simulink model "cruise_control_external_sfun"  (R2013a)
settings: Solver=ode1  StartTime=0.0  StopTime=inf  FixedStep=0.1  RelTol=1e-3
PreLoadFcn:
  | load('cruise_control_external.mat')
undefined symbols (not defined in the file): Ki, Kp
libraries: utility x1
settings Model: Creator=luca  LastModifiedBy=luca

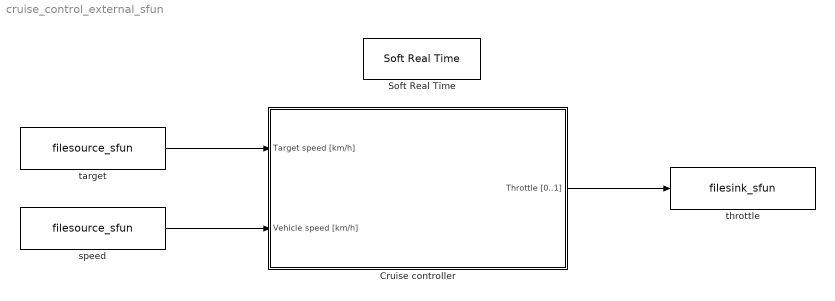
== system cruise_control_external_sfun ==
  Cruise controller : Subsystem
  Soft Real Time : utility/Soft Real Time  x=1
  speed : S-Function  FunctionName=filesource_sfun  Parameters='speed.txt' 0  EnableBusSupport=off
  target : S-Function  FunctionName=filesource_sfun  Parameters='target.txt' 0  EnableBusSupport=off
  throttle : S-Function  FunctionName=filesink_sfun  Parameters='throttle.txt'  EnableBusSupport=off
  wires:
  Cruise controller/1(Throttle [0..1]) -> throttle/1
  speed/1 -> Cruise controller/2(Vehicle speed [km/h])
  target/1 -> Cruise controller/1(Target speed [km/h])

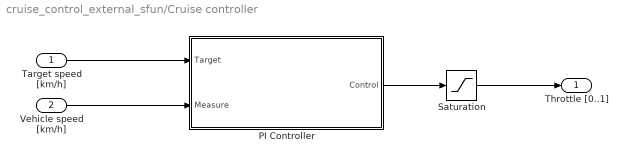
== system cruise_control_external_sfun/Cruise controller ==
  Target speed [km/h] : Inport
  Vehicle speed [km/h] : Inport  Port=2
  PI Controller : Subsystem
  Saturation : Saturate  UpperLimit=1  LowerLimit=0
  Throttle [0..1] : Outport
  wires:
  Vehicle speed [km/h]/1 -> PI Controller/2(Measure)
  PI Controller/1(Control) -> Saturation/1
  Saturation/1 -> Throttle [0..1]/1
  Target speed [km/h]/1 -> PI Controller/1(Target)

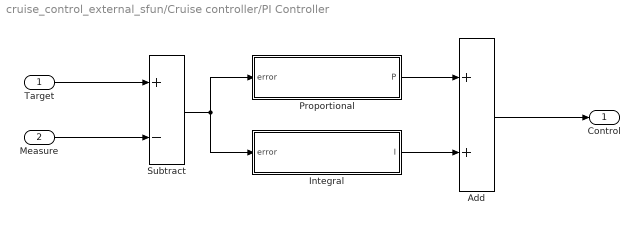
== system cruise_control_external_sfun/Cruise controller/PI Controller ==
  Target : Inport
  Measure : Inport  Port=2
  Add : Sum
  Integral : Subsystem
  Proportional : Subsystem
  Subtract : Sum  Inputs=+-
  Control : Outport
  wires:
  Subtract/1 -> Integral/1(error), Proportional/1(error)
  Target/1 -> Subtract/1
  Measure/1 -> Subtract/2
  Integral/1(I) -> Add/2
  Proportional/1(P) -> Add/1
  Add/1 -> Control/1

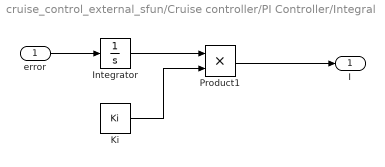
== system cruise_control_external_sfun/Cruise controller/PI Controller/Integral ==
  error : Inport
  Integrator : Integrator
  Ki : Constant  Value=Ki
  Product1 : Product
  I : Outport
  wires:
  Ki/1 -> Product1/2
  Integrator/1 -> Product1/1
  Product1/1 -> I/1
  error/1 -> Integrator/1

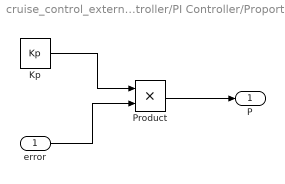
== system cruise_control_external_sfun/Cruise controller/PI Controller/Proportional ==
  error : Inport
  Kp : Constant  Value=Kp
  Product : Product
  P : Outport
  wires:
  Kp/1 -> Product/1
  Product/1 -> P/1
  error/1 -> Product/2
